simulink model "ControlDataSSM0709"  (R2023b)
settings: Solver=FixedStepAuto  StartTime=0.0  StopTime=inf  FixedStep=0.01  RelTol=1e-3
undefined symbols (not defined in the file): Down, Pull
libraries: simulink x39, speedgoatlib_IO691 x23, canmsglib x22, slrealtimeutilitieslib x1, slrealtimeiplib x1
(part 2 of 2)

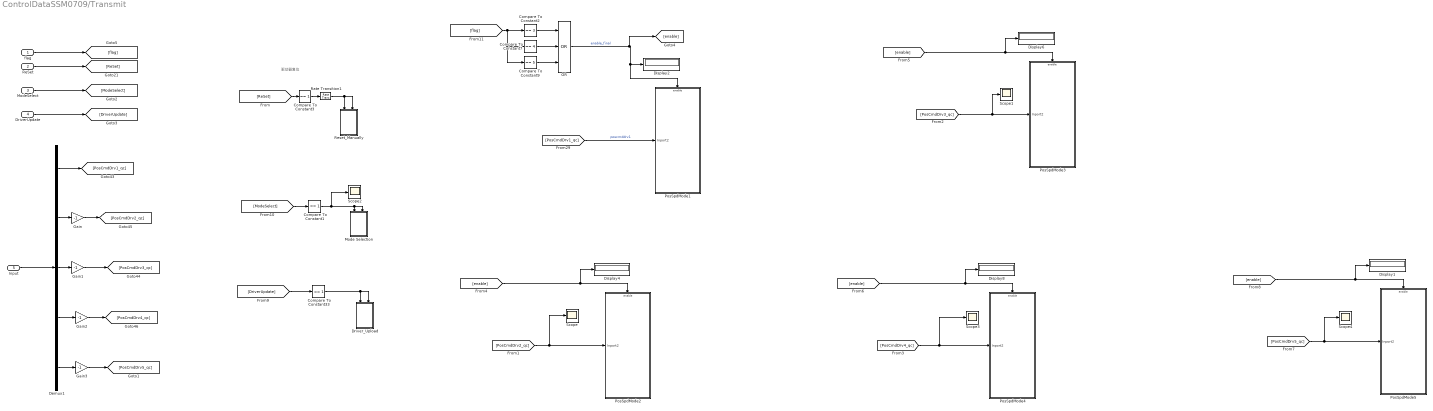
== system ControlDataSSM0709/Transmit ==
  note: 驱动器复位
  flag : Inport
  ReSet : Inport  Port=2
  ModeSelect : Inport  Port=3
  DriverUpdate : Inport  Port=4
  Input : Inport  Port=5
  Compare To Constant1 : simulink/Logic and Bit Operations/Compare To Constant  relop===  const=1  OutDataTypeStr=boolean
  Compare To Constant2 : simulink/Logic and Bit Operations/Compare To Constant  relop===  const=3  OutDataTypeStr=boolean
  Compare To Constant3 : simulink/Logic and Bit Operations/Compare To Constant  relop===  const=1  OutDataTypeStr=boolean
  Compare To Constant33 : simulink/Logic and Bit Operations/Compare To Constant  relop===  const=1  OutDataTypeStr=boolean
  Compare To Constant7 : simulink/Logic and Bit Operations/Compare To Constant  relop===  const=4  OutDataTypeStr=boolean
  Compare To Constant9 : simulink/Logic and Bit Operations/Compare To Constant  relop===  const=5  OutDataTypeStr=boolean
  Demux1 : Demux  Outputs=5
  Display{1..2,4,6,8} (5 alike) : Display
  Driver_Upload : Subsystem
  Gain{,1..3} (4 alike) : Gain  Gain=-1
  Mode Selection : Subsystem  ScheduleAs=Aperiodic partition  PartitionName=TEMP_PRECOMP_PARTITION_NAME_MessageTriggeredSubsystem
  OR : Logic  Operator=OR  Inputs=3  IconShape=distinctive  AllPortsSameDT=off  OutDataTypeStr=boolean
  PosSpdMode1 : Subsystem
  PosSpdMode2 : Subsystem
  PosSpdMode3 : Subsystem
  PosSpdMode4 : Subsystem
  PosSpdMode5 : Subsystem
  Rate Transition1 : RateTransition  OutPortSampleTime=1
  Reset_Manually : Subsystem
  Scope{,1..4} (5 alike) : Scope
  wires:
  Compare To Constant1/1 -> Mode Selection/Trigger, Mode Selection/Enable, Scope2/1
  OR/1 -> [enable], PosSpdMode1/Enable, Display2/1  "enable_final"
  [ReSet] -> Compare To Constant3/1
  Compare To Constant3/1 -> Rate Transition1/1
  Rate Transition1/1 -> Reset_Manually/Trigger, Reset_Manually/Enable
  Demux1/1 -> [PosCmdDrv1_qc]
  Demux1/3 -> Gain1/1
  Demux1/4 -> Gain2/1
  Input/1 -> Demux1/1
  Demux1/2 -> Gain/1
  ReSet/1 -> [ReSet]
  [enable] -> Display4/1, PosSpdMode2/Enable
  [enable] -> Display6/1, PosSpdMode3/Enable
  [enable] -> Display8/1, PosSpdMode4/Enable
  Compare To Constant33/1 -> Driver_Upload/Trigger, Driver_Upload/Enable
  Gain/1 -> [PosCmdDrv2_qc]
  Gain1/1 -> [PosCmdDrv3_qc]
  Gain2/1 -> [PosCmdDrv4_qc]
  [PosCmdDrv1_qc] -> PosSpdMode1/1(Inport2)  "poscmddrv1"
  [PosCmdDrv3_qc] -> Scope1/1, PosSpdMode3/1(Inport2)
  [PosCmdDrv2_qc] -> Scope/1, PosSpdMode2/1(Inport2)
  [PosCmdDrv4_qc] -> Scope3/1, PosSpdMode4/1(Inport2)
  [enable] -> Display1/1, PosSpdMode5/Enable
  [PosCmdDrv5_qc] -> Scope4/1, PosSpdMode5/1(Inport2)
  Demux1/5 -> Gain3/1
  Gain3/1 -> [PosCmdDrv5_qc]
  ModeSelect/1 -> [ModeSelect]
  DriverUpdate/1 -> [DriverUpdate]
  [ModeSelect] -> Compare To Constant1/1
  [DriverUpdate] -> Compare To Constant33/1
  flag/1 -> [flag]
  [flag] -> Compare To Constant9/1, Compare To Constant7/1, Compare To Constant2/1
  Compare To Constant2/1 -> OR/1
  Compare To Constant7/1 -> OR/2
  Compare To Constant9/1 -> OR/3

== system ControlDataSSM0709/Displacement_mode_flag=2/Subsystem1 ==
  position_in : Inport
  Enable : EnablePort
  position_out : Outport
  wires:
  position_in/1 -> position_out/1

== system ControlDataSSM0709/Displacement_mode_flag=2/Subsystem2 ==
  position_in : Inport
  Enable : EnablePort
  position_out : Outport
  wires:
  position_in/1 -> position_out/1

== system ControlDataSSM0709/Displacement_mode_flag=2/Subsystem3 ==
  position_in : Inport
  Enable : EnablePort
  position_out : Outport
  wires:
  position_in/1 -> position_out/1

== system ControlDataSSM0709/Displacement_mode_flag=2/Subsystem5 ==
  position_in : Inport
  Enable : EnablePort
  position_out : Outport
  wires:
  position_in/1 -> position_out/1

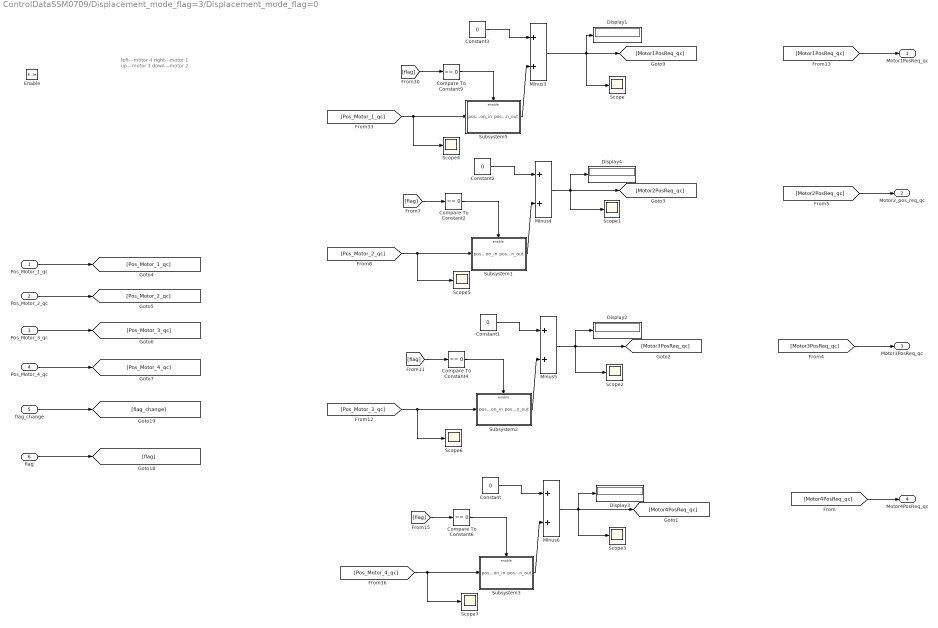
== system ControlDataSSM0709/Displacement_mode_flag=3/Displacement_mode_flag=0 ==
  note: left---motor 4
      | right---motor 1
      | up---motor 3
      | down---motor 2
  Pos_Motor_1_qc : Inport
  Pos_Motor_2_qc : Inport  Port=2
  Pos_Motor_3_qc : Inport  Port=3
  Pos_Motor_4_qc : Inport  Port=4
  flag_change : Inport  Port=5
  flag : Inport  Port=6
  Enable : EnablePort
  Compare To Constant{2,4,6,9} (4 alike) : simulink/Logic and Bit Operations/Compare To Constant  relop===  const=0  OutDataTypeStr=boolean
  Constant{,1..3} (4 alike) : Constant  Value=0
  Display{1..4} (4 alike) : Display
  Minus{3..6} (4 alike) : Sum
  Scope{,1..7} (8 alike) : Scope
  Subsystem1 : Subsystem
  Subsystem2 : Subsystem
  Subsystem3 : Subsystem
  Subsystem5 : Subsystem
  Motor1PosReq_qc : Outport
  Motor2_pos_req_qc : Outport  Port=2
  Motor3PosReq_qc : Outport  Port=3
  Motor4PosReq_qc : Outport  Port=4
  wires:
  Pos_Motor_4_qc/1 -> [Pos_Motor_4_qc]
  Pos_Motor_3_qc/1 -> [Pos_Motor_3_qc]
  Pos_Motor_2_qc/1 -> [Pos_Motor_2_qc]
  Pos_Motor_1_qc/1 -> [Pos_Motor_1_qc]
  flag/1 -> [flag]
  flag_change/1 -> [flag_change]
  [Pos_Motor_1_qc] -> Scope4/1, Subsystem5/1(position_in)
  [flag] -> Compare To Constant9/1
  Compare To Constant9/1 -> Subsystem5/Enable
  Constant3/1 -> Minus3/1
  Minus3/1 -> [Motor1PosReq_qc], Scope/1, Display1/1
  Subsystem5/1(position_out) -> Minus3/2
  Constant2/1 -> Minus4/1
  Compare To Constant2/1 -> Subsystem1/Enable
  [Pos_Motor_2_qc] -> Scope5/1, Subsystem1/1(position_in)
  Minus4/1 -> [Motor2PosReq_qc], Scope1/1, Display4/1
  Subsystem1/1(position_out) -> Minus4/2
  [flag] -> Compare To Constant2/1
  [flag] -> Compare To Constant4/1
  Subsystem2/1(position_out) -> Minus5/2
  Minus5/1 -> [Motor3PosReq_qc], Scope2/1, Display2/1
  Compare To Constant4/1 -> Subsystem2/Enable
  [Pos_Motor_3_qc] -> Scope6/1, Subsystem2/1(position_in)
  Constant1/1 -> Minus5/1
  [flag] -> Compare To Constant6/1
  Subsystem3/1(position_out) -> Minus6/2
  Minus6/1 -> [Motor4PosReq_qc], Scope3/1, Display3/1
  Compare To Constant6/1 -> Subsystem3/Enable
  [Pos_Motor_4_qc] -> Scope7/1, Subsystem3/1(position_in)
  Constant/1 -> Minus6/1
  [Motor4PosReq_qc] -> Motor4PosReq_qc/1
  [Motor3PosReq_qc] -> Motor3PosReq_qc/1
  [Motor2PosReq_qc] -> Motor2_pos_req_qc/1
  [Motor1PosReq_qc] -> Motor1PosReq_qc/1

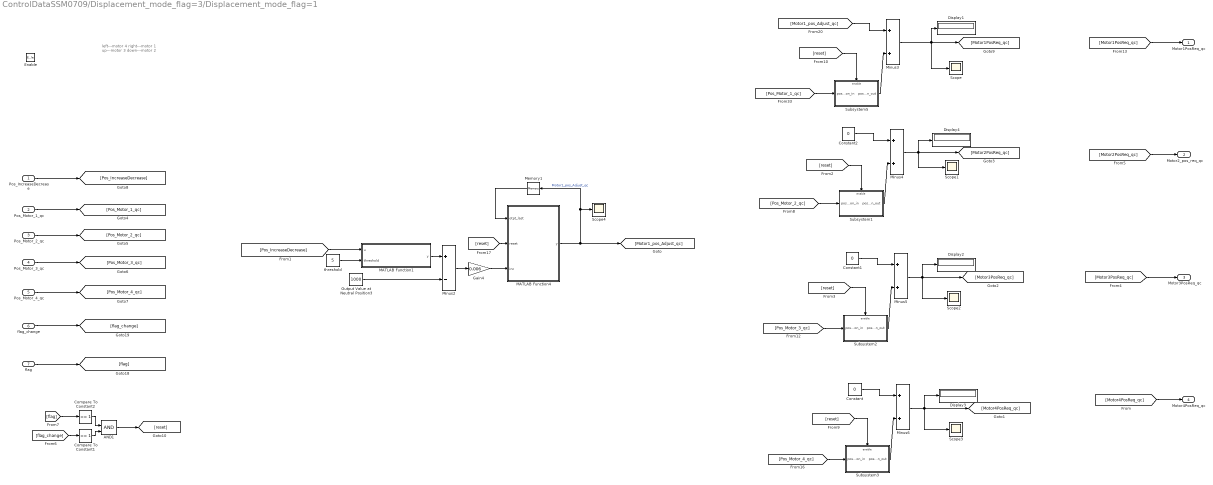
== system ControlDataSSM0709/Displacement_mode_flag=3/Displacement_mode_flag=1 ==
  note: left---motor 4
      | right---motor 1
      | up---motor 3
      | down---motor 2
  Pos_IncreaseDecrease : Inport
  Pos_Motor_1_qc : Inport  Port=2
  Pos_Motor_2_qc : Inport  Port=3
  Pos_Motor_3_qc : Inport  Port=4
  Pos_Motor_4_qc : Inport  Port=5
  flag_change : Inport  Port=6
  flag : Inport  Port=7
  Enable : EnablePort
  AND1 : Logic  IconShape=distinctive  AllPortsSameDT=off  OutDataTypeStr=boolean
  Compare To Constant1 : simulink/Logic and Bit Operations/Compare To Constant  relop===  const=1  OutDataTypeStr=boolean
  Compare To Constant2 : simulink/Logic and Bit Operations/Compare To Constant  relop===  const=1  OutDataTypeStr=boolean
  Constant : Constant  Value=0
  Constant1 : Constant  Value=0
  Constant2 : Constant  Value=0
  Display{1..4} (4 alike) : Display
  Gain4 : Gain  Gain=0.006
  MATLAB Function1 : MATLAB Function  TreatAsAtomicUnit=on
  MATLAB Function4 : MATLAB Function  TreatAsAtomicUnit=on
  Memory1 : Memory
  Minus2 : Sum  Inputs=+-
  Minus{3..6} (4 alike) : Sum
  Output Value at Neutral Position3 : Constant  Value=1000
  Scope{,1..4} (5 alike) : Scope
  Subsystem1 : Subsystem
  Subsystem2 : Subsystem
  Subsystem3 : Subsystem
  Subsystem5 : Subsystem
  threshold : Constant  Value=5
  Motor1PosReq_qc : Outport
  Motor2_pos_req_qc : Outport  Port=2
  Motor3PosReq_qc : Outport  Port=3
  Motor4PosReq_qc : Outport  Port=4
  wires:
  Minus2/1 -> Gain4/1
  [Pos_IncreaseDecrease] -> MATLAB Function1/1(u)
  MATLAB Function1/1(y) -> Minus2/1
  threshold/1 -> MATLAB Function1/2(threshold)
  Output Value at Neutral Position3/1 -> Minus2/2
  Pos_Motor_4_qc/1 -> [Pos_Motor_4_qc]
  Pos_Motor_3_qc/1 -> [Pos_Motor_3_qc]
  Pos_Motor_2_qc/1 -> [Pos_Motor_2_qc]
  Pos_Motor_1_qc/1 -> [Pos_Motor_1_qc]
  flag/1 -> [flag]
  flag_change/1 -> [flag_change]
  [Pos_Motor_1_qc] -> Subsystem5/1(position_in)
  [reset] -> Subsystem5/Enable
  [Motor1_pos_Adjust_qc] -> Minus3/1
  Minus3/1 -> [Motor1PosReq_qc], Scope/1, Display1/1
  Subsystem5/1(position_out) -> Minus3/2
  Constant2/1 -> Minus4/1
  [reset] -> Subsystem1/Enable
  [Pos_Motor_2_qc] -> Subsystem1/1(position_in)
  Minus4/1 -> [Motor2PosReq_qc], Scope1/1, Display4/1
  Subsystem1/1(position_out) -> Minus4/2
  Subsystem2/1(position_out) -> Minus5/2
  Minus5/1 -> [Motor3PosReq_qc], Scope2/1, Display2/1
  [reset] -> Subsystem2/Enable
  [Pos_Motor_3_qc] -> Subsystem2/1(position_in)
  Constant1/1 -> Minus5/1
  Subsystem3/1(position_out) -> Minus6/2
  Minus6/1 -> [Motor4PosReq_qc], Scope3/1, Display3/1
  [reset] -> Subsystem3/Enable
  [Pos_Motor_4_qc] -> Subsystem3/1(position_in)
  Constant/1 -> Minus6/1
  Gain4/1 -> MATLAB Function4/3(inc)
  Pos_IncreaseDecrease/1 -> [Pos_IncreaseDecrease]
  [Motor4PosReq_qc] -> Motor4PosReq_qc/1
  [Motor3PosReq_qc] -> Motor3PosReq_qc/1
  [Motor2PosReq_qc] -> Motor2_pos_req_qc/1
  [Motor1PosReq_qc] -> Motor1PosReq_qc/1
  [reset] -> MATLAB Function4/2(reset)
  Memory1/1 -> MATLAB Function4/1(otpt_last)
  MATLAB Function4/1(y) -> [Motor1_pos_Adjust_qc], Memory1/1, Scope4/1  "Motor1_pos_Adjust_qc"
  Compare To Constant1/1 -> AND1/2
  [flag_change] -> Compare To Constant1/1
  Compare To Constant2/1 -> AND1/1
  [flag] -> Compare To Constant2/1
  AND1/1 -> [reset]

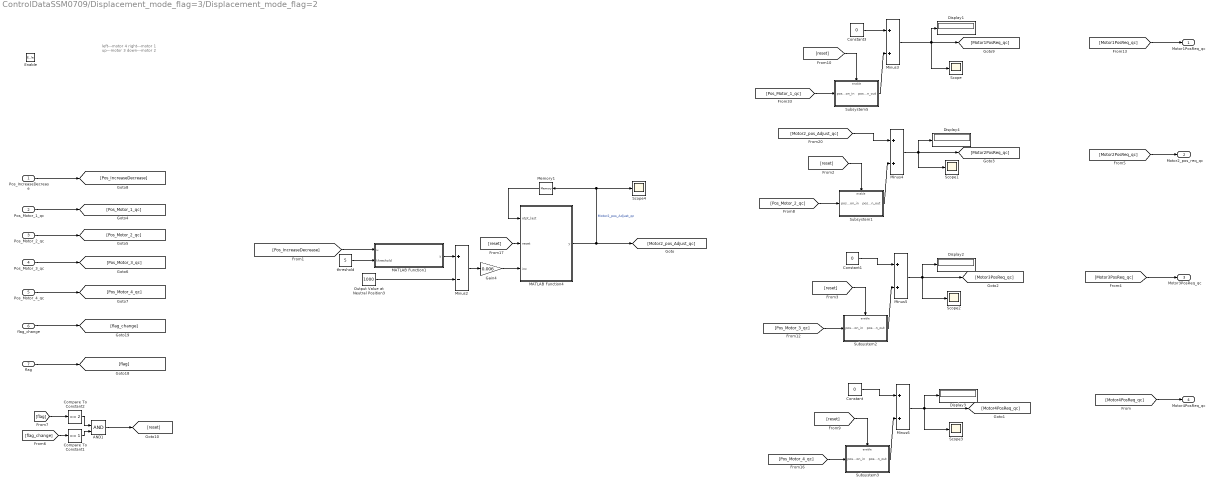
== system ControlDataSSM0709/Displacement_mode_flag=3/Displacement_mode_flag=2 ==
  note: left---motor 4
      | right---motor 1
      | up---motor 3
      | down---motor 2
  Pos_IncreaseDecrease : Inport
  Pos_Motor_1_qc : Inport  Port=2
  Pos_Motor_2_qc : Inport  Port=3
  Pos_Motor_3_qc : Inport  Port=4
  Pos_Motor_4_qc : Inport  Port=5
  flag_change : Inport  Port=6
  flag : Inport  Port=7
  Enable : EnablePort
  AND1 : Logic  IconShape=distinctive  AllPortsSameDT=off  OutDataTypeStr=boolean
  Compare To Constant1 : simulink/Logic and Bit Operations/Compare To Constant  relop===  const=1  OutDataTypeStr=boolean
  Compare To Constant2 : simulink/Logic and Bit Operations/Compare To Constant  relop===  const=2  OutDataTypeStr=boolean
  Constant : Constant  Value=0
  Constant1 : Constant  Value=0
  Constant3 : Constant  Value=0
  Display{1..4} (4 alike) : Display
  Gain4 : Gain  Gain=0.006
  MATLAB Function1 : MATLAB Function  TreatAsAtomicUnit=on
  MATLAB Function4 : MATLAB Function  TreatAsAtomicUnit=on
  Memory1 : Memory
  Minus2 : Sum  Inputs=+-
  Minus{3..6} (4 alike) : Sum
  Output Value at Neutral Position3 : Constant  Value=1000
  Scope{,1..4} (5 alike) : Scope
  Subsystem1 : Subsystem
  Subsystem2 : Subsystem
  Subsystem3 : Subsystem
  Subsystem5 : Subsystem
  threshold : Constant  Value=5
  Motor1PosReq_qc : Outport
  Motor2_pos_req_qc : Outport  Port=2
  Motor3PosReq_qc : Outport  Port=3
  Motor4PosReq_qc : Outport  Port=4
  wires:
  Minus2/1 -> Gain4/1
  [Pos_IncreaseDecrease] -> MATLAB Function1/1(u)
  MATLAB Function1/1(y) -> Minus2/1
  threshold/1 -> MATLAB Function1/2(threshold)
  Output Value at Neutral Position3/1 -> Minus2/2
  Pos_Motor_4_qc/1 -> [Pos_Motor_4_qc]
  Pos_Motor_3_qc/1 -> [Pos_Motor_3_qc]
  Pos_Motor_2_qc/1 -> [Pos_Motor_2_qc]
  Pos_Motor_1_qc/1 -> [Pos_Motor_1_qc]
  flag/1 -> [flag]
  flag_change/1 -> [flag_change]
  [Pos_Motor_1_qc] -> Subsystem5/1(position_in)
  [reset] -> Subsystem5/Enable
  Minus3/1 -> [Motor1PosReq_qc], Scope/1, Display1/1
  Subsystem5/1(position_out) -> Minus3/2
  [Motor2_pos_Adjust_qc] -> Minus4/1
  [reset] -> Subsystem1/Enable
  [Pos_Motor_2_qc] -> Subsystem1/1(position_in)
  Minus4/1 -> [Motor2PosReq_qc], Scope1/1, Display4/1
  Subsystem1/1(position_out) -> Minus4/2
  Subsystem2/1(position_out) -> Minus5/2
  Minus5/1 -> [Motor3PosReq_qc], Scope2/1, Display2/1
  [reset] -> Subsystem2/Enable
  [Pos_Motor_3_qc] -> Subsystem2/1(position_in)
  Constant1/1 -> Minus5/1
  Subsystem3/1(position_out) -> Minus6/2
  Minus6/1 -> [Motor4PosReq_qc], Scope3/1, Display3/1
  [reset] -> Subsystem3/Enable
  [Pos_Motor_4_qc] -> Subsystem3/1(position_in)
  Constant/1 -> Minus6/1
  Gain4/1 -> MATLAB Function4/3(inc)
  Pos_IncreaseDecrease/1 -> [Pos_IncreaseDecrease]
  [Motor4PosReq_qc] -> Motor4PosReq_qc/1
  [Motor3PosReq_qc] -> Motor3PosReq_qc/1
  [Motor2PosReq_qc] -> Motor2_pos_req_qc/1
  [Motor1PosReq_qc] -> Motor1PosReq_qc/1
  Constant3/1 -> Minus3/1
  Compare To Constant1/1 -> AND1/2
  [flag_change] -> Compare To Constant1/1
  Compare To Constant2/1 -> AND1/1
  [flag] -> Compare To Constant2/1
  AND1/1 -> [reset]
  [reset] -> MATLAB Function4/2(reset)
  Memory1/1 -> MATLAB Function4/1(otpt_last)
  MATLAB Function4/1(y) -> Scope4/1, Memory1/1, [Motor2_pos_Adjust_qc]  "Motor2_pos_Adjust_qc"

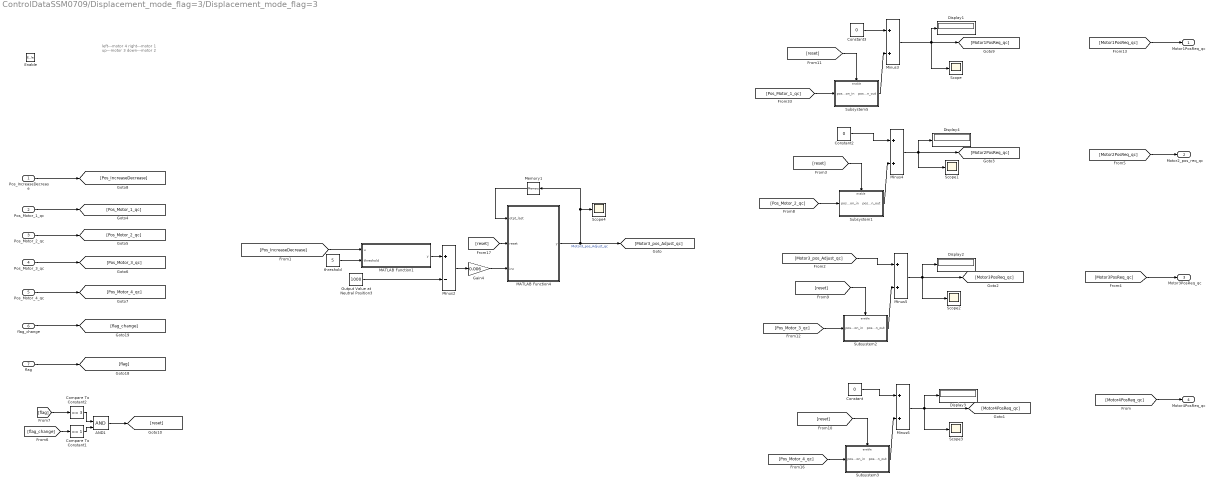
== system ControlDataSSM0709/Displacement_mode_flag=3/Displacement_mode_flag=3 ==
  note: left---motor 4
      | right---motor 1
      | up---motor 3
      | down---motor 2
  Pos_IncreaseDecrease : Inport
  Pos_Motor_1_qc : Inport  Port=2
  Pos_Motor_2_qc : Inport  Port=3
  Pos_Motor_3_qc : Inport  Port=4
  Pos_Motor_4_qc : Inport  Port=5
  flag_change : Inport  Port=6
  flag : Inport  Port=7
  Enable : EnablePort
  AND1 : Logic  IconShape=distinctive  AllPortsSameDT=off  OutDataTypeStr=boolean
  Compare To Constant1 : simulink/Logic and Bit Operations/Compare To Constant  relop===  const=1  OutDataTypeStr=boolean
  Compare To Constant2 : simulink/Logic and Bit Operations/Compare To Constant  relop===  const=3  OutDataTypeStr=boolean
  Constant : Constant  Value=0
  Constant2 : Constant  Value=0
  Constant3 : Constant  Value=0
  Display{1..4} (4 alike) : Display
  Gain4 : Gain  Gain=0.006
  MATLAB Function1 : MATLAB Function  TreatAsAtomicUnit=on
  MATLAB Function4 : MATLAB Function  TreatAsAtomicUnit=on
  Memory1 : Memory
  Minus2 : Sum  Inputs=+-
  Minus{3..6} (4 alike) : Sum
  Output Value at Neutral Position3 : Constant  Value=1000
  Scope{,1..4} (5 alike) : Scope
  Subsystem1 : Subsystem
  Subsystem2 : Subsystem
  Subsystem3 : Subsystem
  Subsystem5 : Subsystem
  threshold : Constant  Value=5
  Motor1PosReq_qc : Outport
  Motor2_pos_req_qc : Outport  Port=2
  Motor3PosReq_qc : Outport  Port=3
  Motor4PosReq_qc : Outport  Port=4
  wires:
  Minus2/1 -> Gain4/1
  [Pos_IncreaseDecrease] -> MATLAB Function1/1(u)
  MATLAB Function1/1(y) -> Minus2/1
  threshold/1 -> MATLAB Function1/2(threshold)
  Output Value at Neutral Position3/1 -> Minus2/2
  Pos_Motor_4_qc/1 -> [Pos_Motor_4_qc]
  Pos_Motor_3_qc/1 -> [Pos_Motor_3_qc]
  Pos_Motor_2_qc/1 -> [Pos_Motor_2_qc]
  Pos_Motor_1_qc/1 -> [Pos_Motor_1_qc]
  flag/1 -> [flag]
  flag_change/1 -> [flag_change]
  [Pos_Motor_1_qc] -> Subsystem5/1(position_in)
  [reset] -> Subsystem5/Enable
  Minus3/1 -> [Motor1PosReq_qc], Scope/1, Display1/1
  Subsystem5/1(position_out) -> Minus3/2
  Constant2/1 -> Minus4/1
  [reset] -> Subsystem1/Enable
  [Pos_Motor_2_qc] -> Subsystem1/1(position_in)
  Minus4/1 -> [Motor2PosReq_qc], Scope1/1, Display4/1
  Subsystem1/1(position_out) -> Minus4/2
  Subsystem2/1(position_out) -> Minus5/2
  Minus5/1 -> [Motor3PosReq_qc], Scope2/1, Display2/1
  [reset] -> Subsystem2/Enable
  [Pos_Motor_3_qc] -> Subsystem2/1(position_in)
  [Motor3_pos_Adjust_qc] -> Minus5/1
  Subsystem3/1(position_out) -> Minus6/2
  Minus6/1 -> [Motor4PosReq_qc], Scope3/1, Display3/1
  [reset] -> Subsystem3/Enable
  [Pos_Motor_4_qc] -> Subsystem3/1(position_in)
  Constant/1 -> Minus6/1
  Gain4/1 -> MATLAB Function4/3(inc)
  Pos_IncreaseDecrease/1 -> [Pos_IncreaseDecrease]
  [Motor4PosReq_qc] -> Motor4PosReq_qc/1
  [Motor3PosReq_qc] -> Motor3PosReq_qc/1
  [Motor2PosReq_qc] -> Motor2_pos_req_qc/1
  [Motor1PosReq_qc] -> Motor1PosReq_qc/1
  Constant3/1 -> Minus3/1
  Compare To Constant1/1 -> AND1/2
  [flag_change] -> Compare To Constant1/1
  [flag] -> Compare To Constant2/1
  Compare To Constant2/1 -> AND1/1
  AND1/1 -> [reset]
  [reset] -> MATLAB Function4/2(reset)
  Memory1/1 -> MATLAB Function4/1(otpt_last)
  MATLAB Function4/1(y) -> Scope4/1, Memory1/1, [Motor3_pos_Adjust_qc]  "Motor3_pos_Adjust_qc"

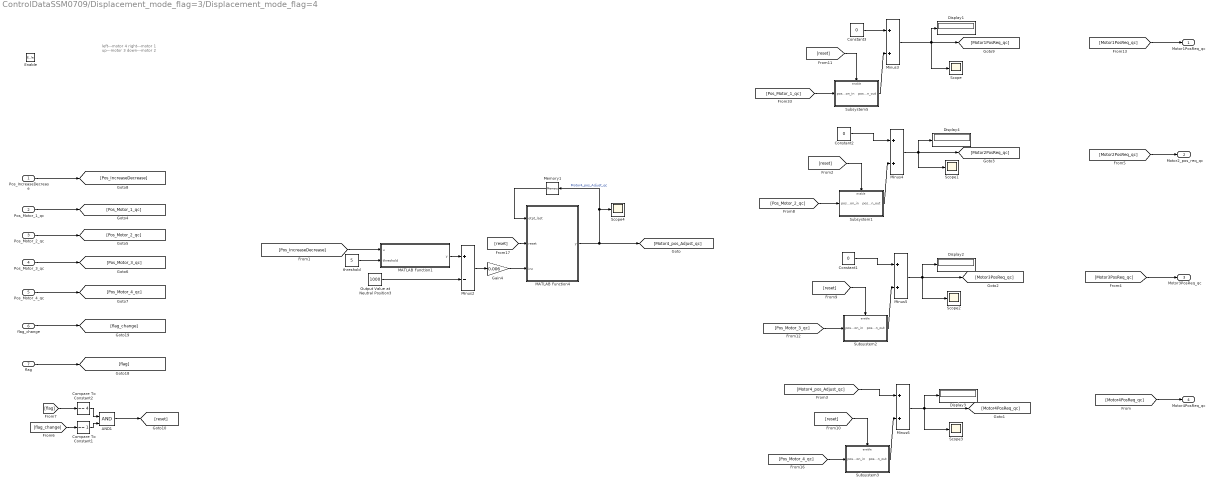
== system ControlDataSSM0709/Displacement_mode_flag=3/Displacement_mode_flag=4 ==
  note: left---motor 4
      | right---motor 1
      | up---motor 3
      | down---motor 2
  Pos_IncreaseDecrease : Inport
  Pos_Motor_1_qc : Inport  Port=2
  Pos_Motor_2_qc : Inport  Port=3
  Pos_Motor_3_qc : Inport  Port=4
  Pos_Motor_4_qc : Inport  Port=5
  flag_change : Inport  Port=6
  flag : Inport  Port=7
  Enable : EnablePort
  AND1 : Logic  IconShape=distinctive  AllPortsSameDT=off  OutDataTypeStr=boolean
  Compare To Constant1 : simulink/Logic and Bit Operations/Compare To Constant  relop===  const=1  OutDataTypeStr=boolean
  Compare To Constant2 : simulink/Logic and Bit Operations/Compare To Constant  relop===  const=4  OutDataTypeStr=boolean
  Constant1 : Constant  Value=0
  Constant2 : Constant  Value=0
  Constant3 : Constant  Value=0
  Display{1..4} (4 alike) : Display
  Gain4 : Gain  Gain=0.006
  MATLAB Function1 : MATLAB Function  TreatAsAtomicUnit=on
  MATLAB Function4 : MATLAB Function  TreatAsAtomicUnit=on
  Memory1 : Memory
  Minus2 : Sum  Inputs=+-
  Minus{3..6} (4 alike) : Sum
  Output Value at Neutral Position3 : Constant  Value=1000
  Scope{,1..4} (5 alike) : Scope
  Subsystem1 : Subsystem
  Subsystem2 : Subsystem
  Subsystem3 : Subsystem
  Subsystem5 : Subsystem
  threshold : Constant  Value=5
  Motor1PosReq_qc : Outport
  Motor2_pos_req_qc : Outport  Port=2
  Motor3PosReq_qc : Outport  Port=3
  Motor4PosReq_qc : Outport  Port=4
  wires:
  Constant3/1 -> Minus3/1
  [Motor1PosReq_qc] -> Motor1PosReq_qc/1
  [Motor2PosReq_qc] -> Motor2_pos_req_qc/1
  [Motor3PosReq_qc] -> Motor3PosReq_qc/1
  [Motor4PosReq_qc] -> Motor4PosReq_qc/1
  Pos_IncreaseDecrease/1 -> [Pos_IncreaseDecrease]
  Gain4/1 -> MATLAB Function4/3(inc)
  [Motor4_pos_Adjust_qc] -> Minus6/1
  [Pos_Motor_4_qc] -> Subsystem3/1(position_in)
  [reset] -> Subsystem3/Enable
  Minus6/1 -> Display3/1, Scope3/1, [Motor4PosReq_qc]
  Subsystem3/1(position_out) -> Minus6/2
  Constant1/1 -> Minus5/1
  [Pos_Motor_3_qc] -> Subsystem2/1(position_in)
  [reset] -> Subsystem2/Enable
  Minus5/1 -> Display2/1, Scope2/1, [Motor3PosReq_qc]
  Subsystem2/1(position_out) -> Minus5/2
  Subsystem1/1(position_out) -> Minus4/2
  Minus4/1 -> Display4/1, Scope1/1, [Motor2PosReq_qc]
  [Pos_Motor_2_qc] -> Subsystem1/1(position_in)
  [reset] -> Subsystem1/Enable
  Constant2/1 -> Minus4/1
  Subsystem5/1(position_out) -> Minus3/2
  Minus3/1 -> Display1/1, Scope/1, [Motor1PosReq_qc]
  [reset] -> Subsystem5/Enable
  [Pos_Motor_1_qc] -> Subsystem5/1(position_in)
  flag_change/1 -> [flag_change]
  flag/1 -> [flag]
  Pos_Motor_1_qc/1 -> [Pos_Motor_1_qc]
  Pos_Motor_2_qc/1 -> [Pos_Motor_2_qc]
  Pos_Motor_3_qc/1 -> [Pos_Motor_3_qc]
  Pos_Motor_4_qc/1 -> [Pos_Motor_4_qc]
  Output Value at Neutral Position3/1 -> Minus2/2
  threshold/1 -> MATLAB Function1/2(threshold)
  MATLAB Function1/1(y) -> Minus2/1
  [Pos_IncreaseDecrease] -> MATLAB Function1/1(u)
  Minus2/1 -> Gain4/1
  [flag_change] -> Compare To Constant1/1
  Compare To Constant2/1 -> AND1/1
  Compare To Constant1/1 -> AND1/2
  [flag] -> Compare To Constant2/1
  AND1/1 -> [reset]
  Memory1/1 -> MATLAB Function4/1(otpt_last)
  [reset] -> MATLAB Function4/2(reset)
  MATLAB Function4/1(y) -> Scope4/1, Memory1/1, [Motor4_pos_Adjust_qc]  "Motor4_pos_Adjust_qc"

== system ControlDataSSM0709/Transmit/Driver_Upload ==
  Enable : EnablePort  StatesWhenEnabling=reset
  Trigger : TriggerPort  VariantControl=(inherit)  PortDimensions=1
  CAN Pack : canmsglib/CAN Pack  CANdbFile=E:\OneDrive\OneDrive - The Chinese University of Hong Kong\文档\Research\SRIL\12nd\Experiment\Simulink\RoboModule0729.dbc  MsgList=Configuration_all  MsgName=Configuration_all  MsgIDType=Standard (11-bit identifier)  MsgIdentifier=10  MsgLength=8  Remote=off  ApplyMinMax=off  BusOutput=off  SignalInfo={'Data2','16','8','BE','unsigned','Standard','0','1','0','-Inf','Inf';'Data3','24','8','BE','unsigned','Standard','0','1','0','-Inf','Inf';'Data4','32','8','BE','unsigned','Standard','0','1','0','-Inf','Inf';'Data5','40','8','BE','unsigned','Standard','0','1','0','-Inf','Inf';'Data6','48','8','BE','unsigned','Standard','0','1','0','-Inf','Inf';'Data7','56','8','BE','unsigned','Standard','0','1','0','-Inf','Inf';'output_cycle_curvelpos','0','8','BE','unsigned','Standard','0','1','0','-Inf','Inf';'output_cycle_others','8','8','BE','unsigned','Standard','0','1','0','-Inf','Inf'}
      settings: DataFormat=CANdb specified signals
  "CAN Write " : speedgoatlib_IO691/CAN Write   moduleType=IO691  id=1  channel=1  canType=CAN (HS)  messageType=CAN (HS)  useBusIn=off  numOfMsg=1  enableInput=off  enableStatusPort=off  ts=-1  initValues=[691 1 -1 0 1 1 0 1 0 0]
      settings: SourceProductName=Simulink Real-Time: Speedgoat I/O Blockset
  Constant4 : Constant  Value=hex2dec('0x55')  OutDataTypeStr=uint8  SampleTime=-1
  Constant5 : Constant  Value=hex2dec('0x64')  OutDataTypeStr=uint8  SampleTime=-1
  Constant6 : Constant  Value=hex2dec('0x00')  OutDataTypeStr=uint8  SampleTime=-1
  wires:
  CAN Pack/1 -> "CAN Write "/1
  Constant4/1 -> CAN Pack/1, CAN Pack/3, CAN Pack/5, CAN Pack/6, CAN Pack/4, CAN Pack/2
  Constant5/1 -> CAN Pack/7
  Constant6/1 -> CAN Pack/8

== system ControlDataSSM0709/Transmit/Mode Selection ==
  Enable : EnablePort  StatesWhenEnabling=reset
  Trigger : TriggerPort  VariantControl=(inherit)  PortDimensions=1
  CAN Pack : canmsglib/CAN Pack  CANdbFile=E:\Research\SRIL\12nd\Simulink\RoboModule0729.dbc  MsgList=Mode_Selection_all  MsgName=Mode_Selection_all  MsgIDType=Standard (11-bit identifier)  MsgIdentifier=1  MsgLength=8  Remote=off  ApplyMinMax=off  BusOutput=off  SignalInfo={'Data1','8','8','BE','unsigned','Standard','0','1','0','-Inf','Inf';'Data2','16','8','BE','unsigned','Standard','0','1','0','-Inf','Inf';'Data3','24','8','BE','unsigned','Standard','0','1','0','-Inf','Inf';'Data4','32','8','BE','unsigned','Standard','0','1','0','-Inf','Inf';'Data5','40','8','BE','unsigned','Standard','0','1','0','-Inf','Inf';'Data6','48','8','BE','unsigned','Standard','0','1','0','-Inf','Inf';'Data7','56','8','BE','unsigned','Standard','0','1','0','-Inf','Inf';'Mode','0','8','BE','unsigned','Standard','0','1','0','-Inf','Inf'}
      settings: DataFormat=CANdb specified signals
  "CAN Write " : speedgoatlib_IO691/CAN Write   moduleType=IO691  id=1  channel=1  canType=CAN (HS)  messageType=CAN (HS)  useBusIn=off  numOfMsg=1  enableInput=off  enableStatusPort=off  ts=-1  initValues=[691 1 -1 0 1 1 0 1 0 0]
      settings: SourceProductName=Simulink Real-Time: Speedgoat I/O Blockset
  Constant2 : Constant  Value=hex2dec('0x55')  OutDataTypeStr=uint8  SampleTime=-1
  Mode Number1 : Constant  Value=hex2dec('0x04')  OutDataTypeStr=uint8  SampleTime=-1
  wires:
  Constant2/1 -> CAN Pack/1, CAN Pack/3, CAN Pack/5, CAN Pack/6, CAN Pack/7, CAN Pack/4, CAN Pack/2
  CAN Pack/1 -> "CAN Write "/1
  Mode Number1/1 -> CAN Pack/8

== system ControlDataSSM0709/Transmit/PosSpdMode1 ==
  note: R ated Voltage of Motor is 12 V. Supply Voltage is 24 V. Limilation of the temp_pwm is set as 2500.
  Inport2 : Inport
  Enable : EnablePort
  CAN Pack : canmsglib/CAN Pack  CANdbFile=E:\OneDrive\OneDrive - The Chinese University of Hong Kong\文档\Research\SRIL\12nd\Experiment\Simulink\RoboModule0729.dbc  MsgList=Position_Dr1  MsgName=Position_Dr1  MsgIDType=Standard (11-bit identifier)  MsgIdentifier=21  MsgLength=8  Remote=off  ApplyMinMax=off  BusOutput=off  SignalInfo={'Data2','16','8','BE','unsigned','Standard','0','1','0','-Inf','Inf';'Data3','24','8','BE','unsigned','Standard','0','1','0','-Inf','Inf';'temp_position','56','32','BE','signed','Standard','0','1','0','-Inf','Inf';'temp_pwm','8','16','BE','unsigned','Standard','0','1','0','-Inf','Inf'}
      settings: DataFormat=CANdb specified signals
  "CAN Write " : speedgoatlib_IO691/CAN Write   moduleType=IO691  id=1  channel=1  canType=CAN (HS)  messageType=CAN (HS)  useBusIn=off  numOfMsg=1  enableInput=off  enableStatusPort=off  ts=-1  initValues=[691 1 -1 0 1 1 0 1 0 0]
      settings: SourceProductName=Simulink Real-Time: Speedgoat I/O Blockset
  Constant1 : Constant  Value=5000
  Constant3 : Constant  Value=hex2dec('0x55')  OutDataTypeStr=uint8  SampleTime=-1
  wires:
  Constant3/1 -> CAN Pack/2, CAN Pack/1
  Inport2/1 -> CAN Pack/3
  Constant1/1 -> CAN Pack/4
  CAN Pack/1 -> "CAN Write "/1

== system ControlDataSSM0709/Transmit/PosSpdMode2 ==
  note: R ated Voltage of Motor is 12 V. Supply Voltage is 24 V. Limilation of the temp_pwm is set as 2500.
  Inport2 : Inport
  Enable : EnablePort
  CAN Pack : canmsglib/CAN Pack  CANdbFile=E:\Research\SRIL\12nd\Simulink\RoboModule0729.dbc  MsgList=Position_Dr2  MsgName=Position_Dr2  MsgIDType=Standard (11-bit identifier)  MsgIdentifier=37  MsgLength=8  Remote=off  ApplyMinMax=off  BusOutput=off  SignalInfo={'Data2','16','8','BE','unsigned','Standard','0','1','0','-Inf','Inf';'Data3','24','8','BE','unsigned','Standard','0','1','0','-Inf','Inf';'temp_position','56','32','BE','signed','Standard','0','1','0','-Inf','Inf';'temp_pwm','8','16','BE','unsigned','Standard','0','1','0','-Inf','Inf'}
      settings: DataFormat=CANdb specified signals
  "CAN Write " : speedgoatlib_IO691/CAN Write   moduleType=IO691  id=1  channel=1  canType=CAN (HS)  messageType=CAN (HS)  useBusIn=off  numOfMsg=1  enableInput=off  enableStatusPort=off  ts=-1  initValues=[691 1 -1 0 1 1 0 1 0 0]
      settings: SourceProductName=Simulink Real-Time: Speedgoat I/O Blockset
  Constant1 : Constant  Value=5000
  Constant3 : Constant  Value=hex2dec('0x55')  OutDataTypeStr=uint8  SampleTime=-1
  Scope : Scope
  wires:
  CAN Pack/1 -> "CAN Write "/1
  Constant3/1 -> CAN Pack/2, CAN Pack/1
  Inport2/1 -> Scope/1, CAN Pack/3
  Constant1/1 -> CAN Pack/4

== system ControlDataSSM0709/Transmit/PosSpdMode3 ==
  note: R ated Voltage of Motor is 12 V. Supply Voltage is 24 V. Limilation of the temp_pwm is set as 2500.
  Inport2 : Inport
  Enable : EnablePort
  CAN Pack : canmsglib/CAN Pack  CANdbFile=E:\OneDrive\OneDrive - The Chinese University of Hong Kong\文档\Research\SRIL\12nd\Experiment\Simulink\RoboModule0729.dbc  MsgList=Position_Dr3  MsgName=Position_Dr3  MsgIDType=Standard (11-bit identifier)  MsgIdentifier=53  MsgLength=8  Remote=off  ApplyMinMax=off  BusOutput=off  SignalInfo={'Data2','16','8','BE','unsigned','Standard','0','1','0','-Inf','Inf';'Data3','24','8','BE','unsigned','Standard','0','1','0','-Inf','Inf';'temp_position','56','32','BE','signed','Standard','0','1','0','-Inf','Inf';'temp_pwm','8','16','BE','unsigned','Standard','0','1','0','-Inf','Inf'}
      settings: DataFormat=CANdb specified signals
  "CAN Write " : speedgoatlib_IO691/CAN Write   moduleType=IO691  id=1  channel=1  canType=CAN (HS)  messageType=CAN (HS)  useBusIn=off  numOfMsg=1  enableInput=off  enableStatusPort=off  ts=-1  initValues=[691 1 -1 0 1 1 0 1 0 0]
      settings: SourceProductName=Simulink Real-Time: Speedgoat I/O Blockset
  Constant1 : Constant  Value=5000
  Constant3 : Constant  Value=hex2dec('0x55')  OutDataTypeStr=uint8  SampleTime=-1
  wires:
  CAN Pack/1 -> "CAN Write "/1
  Constant3/1 -> CAN Pack/2, CAN Pack/1
  Inport2/1 -> CAN Pack/3
  Constant1/1 -> CAN Pack/4

== system ControlDataSSM0709/Transmit/PosSpdMode4 ==
  note: R ated Voltage of Motor is 12 V. Supply Voltage is 24 V. Limilation of the temp_pwm is set as 2500.
  Inport2 : Inport
  Enable : EnablePort
  CAN Pack : canmsglib/CAN Pack  CANdbFile=E:\OneDrive\OneDrive - The Chinese University of Hong Kong\文档\Research\SRIL\12nd\Experiment\Simulink\RoboModule0729.dbc  MsgList=Position_Dr4  MsgName=Position_Dr4  MsgIDType=Standard (11-bit identifier)  MsgIdentifier=69  MsgLength=8  Remote=off  ApplyMinMax=off  BusOutput=off  SignalInfo={'Data2','16','8','BE','unsigned','Standard','0','1','0','-Inf','Inf';'Data3','24','8','BE','unsigned','Standard','0','1','0','-Inf','Inf';'temp_position','56','32','BE','signed','Standard','0','1','0','-Inf','Inf';'temp_pwm','8','16','BE','unsigned','Standard','0','1','0','-Inf','Inf'}
      settings: DataFormat=CANdb specified signals
  "CAN Write " : speedgoatlib_IO691/CAN Write   moduleType=IO691  id=1  channel=1  canType=CAN (HS)  messageType=CAN (HS)  useBusIn=off  numOfMsg=1  enableInput=off  enableStatusPort=off  ts=-1  initValues=[691 1 -1 0 1 1 0 1 0 0]
      settings: SourceProductName=Simulink Real-Time: Speedgoat I/O Blockset
  Constant1 : Constant  Value=5000
  Constant3 : Constant  Value=hex2dec('0x55')  OutDataTypeStr=uint8  SampleTime=-1
  wires:
  CAN Pack/1 -> "CAN Write "/1
  Constant3/1 -> CAN Pack/2, CAN Pack/1
  Inport2/1 -> CAN Pack/3
  Constant1/1 -> CAN Pack/4

== system ControlDataSSM0709/Transmit/PosSpdMode5 ==
  note: R ated Voltage of Motor is 12 V. Supply Voltage is 24 V. Limilation of the temp_pwm is set as 2500.
  Inport2 : Inport
  Enable : EnablePort
  CAN Pack : canmsglib/CAN Pack  CANdbFile=E:\OneDrive\OneDrive - The Chinese University of Hong Kong\文档\Research\SRIL\12nd\Experiment\Simulink\RoboModule0729.dbc  MsgList=Position_Dr5  MsgName=Position_Dr5  MsgIDType=Standard (11-bit identifier)  MsgIdentifier=85  MsgLength=8  Remote=off  ApplyMinMax=off  BusOutput=off  SignalInfo={'Data2','16','8','BE','unsigned','Standard','0','1','0','-Inf','Inf';'Data3','24','8','BE','unsigned','Standard','0','1','0','-Inf','Inf';'temp_position','56','32','BE','signed','Standard','0','1','0','-Inf','Inf';'temp_pwm','8','16','BE','unsigned','Standard','0','1','0','-Inf','Inf'}
      settings: DataFormat=CANdb specified signals
  "CAN Write " : speedgoatlib_IO691/CAN Write   moduleType=IO691  id=1  channel=1  canType=CAN (HS)  messageType=CAN (HS)  useBusIn=off  numOfMsg=1  enableInput=off  enableStatusPort=off  ts=-1  initValues=[691 1 -1 0 1 1 0 1 0 0]
      settings: SourceProductName=Simulink Real-Time: Speedgoat I/O Blockset
  Constant1 : Constant  Value=5000
  Constant3 : Constant  Value=hex2dec('0x55')  OutDataTypeStr=uint8  SampleTime=-1
  Scope : Scope
  wires:
  CAN Pack/1 -> "CAN Write "/1
  Constant3/1 -> CAN Pack/2, CAN Pack/1
  Inport2/1 -> Scope/1, CAN Pack/3
  Constant1/1 -> CAN Pack/4

== system ControlDataSSM0709/Transmit/Reset_Manually ==
  Enable : EnablePort  StatesWhenEnabling=reset
  Trigger : TriggerPort  VariantControl=(inherit)  PortDimensions=1
  CAN Pack : canmsglib/CAN Pack  CANdbFile=E:\OneDrive\OneDrive - The Chinese University of Hong Kong\文档\Research\SRIL\12nd\Experiment\Simulink\RoboModule0729.dbc  MsgList=Reset_all  MsgName=Reset_all  MsgIDType=Standard (11-bit identifier)  MsgIdentifier=0  MsgLength=8  Remote=off  ApplyMinMax=off  BusOutput=off  SignalInfo={'Data0','0','8','BE','unsigned','Standard','0','1','0','-Inf','Inf';'Data1','8','8','BE','unsigned','Standard','0','1','0','-Inf','Inf';'Data2','16','8','BE','unsigned','Standard','0','1','0','-Inf','Inf';'Data3','24','8','BE','unsigned','Standard','0','1','0','-Inf','Inf';'Data4','32','8','BE','unsigned','Standard','0','1','0','-Inf','Inf';'Data5','40','8','BE','unsigned','Standard','0','1','0','-Inf','Inf';'Data6','48','8','BE','unsigned','Standard','0','1','0','-Inf','Inf';'Data7','56','8','BE','unsigned','Standard','0','1','0','-Inf','Inf'}
      settings: DataFormat=CANdb specified signals
  "CAN Write " : speedgoatlib_IO691/CAN Write   moduleType=IO691  id=1  channel=1  canType=CAN (HS)  messageType=CAN (HS)  useBusIn=off  numOfMsg=1  enableInput=off  enableStatusPort=off  ts=-1  initValues=[691 1 -1 0 1 1 0 1 0 0]
      settings: SourceProductName=Simulink Real-Time: Speedgoat I/O Blockset
  Constant2 : Constant  Value=hex2dec('0x55')  OutDataTypeStr=uint8  SampleTime=-1
  wires:
  CAN Pack/1 -> "CAN Write "/1
  Constant2/1 -> CAN Pack/1, CAN Pack/3, CAN Pack/5, CAN Pack/6, CAN Pack/7, CAN Pack/8, CAN Pack/4, CAN Pack/2

== system ControlDataSSM0709/Displacement_mode_flag=3/Displacement_mode_flag=0/Subsystem1 ==
  position_in : Inport
  Enable : EnablePort
  position_out : Outport
  wires:
  position_in/1 -> position_out/1

== system ControlDataSSM0709/Displacement_mode_flag=3/Displacement_mode_flag=0/Subsystem2 ==
  position_in : Inport
  Enable : EnablePort
  position_out : Outport
  wires:
  position_in/1 -> position_out/1

== system ControlDataSSM0709/Displacement_mode_flag=3/Displacement_mode_flag=0/Subsystem3 ==
  position_in : Inport
  Enable : EnablePort
  position_out : Outport
  wires:
  position_in/1 -> position_out/1

== system ControlDataSSM0709/Displacement_mode_flag=3/Displacement_mode_flag=0/Subsystem5 ==
  position_in : Inport
  Enable : EnablePort
  position_out : Outport
  wires:
  position_in/1 -> position_out/1

== system ControlDataSSM0709/Displacement_mode_flag=3/Displacement_mode_flag=1/Subsystem1 ==
  position_in : Inport
  Enable : EnablePort
  position_out : Outport
  wires:
  position_in/1 -> position_out/1

== system ControlDataSSM0709/Displacement_mode_flag=3/Displacement_mode_flag=1/Subsystem2 ==
  position_in : Inport
  Enable : EnablePort
  position_out : Outport
  wires:
  position_in/1 -> position_out/1

== system ControlDataSSM0709/Displacement_mode_flag=3/Displacement_mode_flag=1/Subsystem3 ==
  position_in : Inport
  Enable : EnablePort
  position_out : Outport
  wires:
  position_in/1 -> position_out/1

== system ControlDataSSM0709/Displacement_mode_flag=3/Displacement_mode_flag=1/Subsystem5 ==
  position_in : Inport
  Enable : EnablePort
  position_out : Outport
  wires:
  position_in/1 -> position_out/1

== system ControlDataSSM0709/Displacement_mode_flag=3/Displacement_mode_flag=2/Subsystem1 ==
  position_in : Inport
  Enable : EnablePort
  position_out : Outport
  wires:
  position_in/1 -> position_out/1

== system ControlDataSSM0709/Displacement_mode_flag=3/Displacement_mode_flag=2/Subsystem2 ==
  position_in : Inport
  Enable : EnablePort
  position_out : Outport
  wires:
  position_in/1 -> position_out/1

== system ControlDataSSM0709/Displacement_mode_flag=3/Displacement_mode_flag=2/Subsystem3 ==
  position_in : Inport
  Enable : EnablePort
  position_out : Outport
  wires:
  position_in/1 -> position_out/1

== system ControlDataSSM0709/Displacement_mode_flag=3/Displacement_mode_flag=2/Subsystem5 ==
  position_in : Inport
  Enable : EnablePort
  position_out : Outport
  wires:
  position_in/1 -> position_out/1

== system ControlDataSSM0709/Displacement_mode_flag=3/Displacement_mode_flag=3/Subsystem1 ==
  position_in : Inport
  Enable : EnablePort
  position_out : Outport
  wires:
  position_in/1 -> position_out/1

== system ControlDataSSM0709/Displacement_mode_flag=3/Displacement_mode_flag=3/Subsystem2 ==
  position_in : Inport
  Enable : EnablePort
  position_out : Outport
  wires:
  position_in/1 -> position_out/1

== system ControlDataSSM0709/Displacement_mode_flag=3/Displacement_mode_flag=3/Subsystem3 ==
  position_in : Inport
  Enable : EnablePort
  position_out : Outport
  wires:
  position_in/1 -> position_out/1

== system ControlDataSSM0709/Displacement_mode_flag=3/Displacement_mode_flag=3/Subsystem5 ==
  position_in : Inport
  Enable : EnablePort
  position_out : Outport
  wires:
  position_in/1 -> position_out/1

== system ControlDataSSM0709/Displacement_mode_flag=3/Displacement_mode_flag=4/Subsystem1 ==
  position_in : Inport
  Enable : EnablePort
  position_out : Outport
  wires:
  position_in/1 -> position_out/1

== system ControlDataSSM0709/Displacement_mode_flag=3/Displacement_mode_flag=4/Subsystem2 ==
  position_in : Inport
  Enable : EnablePort
  position_out : Outport
  wires:
  position_in/1 -> position_out/1

== system ControlDataSSM0709/Displacement_mode_flag=3/Displacement_mode_flag=4/Subsystem3 ==
  position_in : Inport
  Enable : EnablePort
  position_out : Outport
  wires:
  position_in/1 -> position_out/1

== system ControlDataSSM0709/Displacement_mode_flag=3/Displacement_mode_flag=4/Subsystem5 ==
  position_in : Inport
  Enable : EnablePort
  position_out : Outport
  wires:
  position_in/1 -> position_out/1

== matlab function ControlDataSSM0709/Displacement_mode_flag=2/RandomControlSequence ==
  settings: updateMethod=DISCRETE
  data: disMotor1 output; disMotor2 output; t input; y_axis data_store_memory; z_axis data_store_memory; disMotor3 output; disMotor4 output; ins output; gain input; zMotor output; yMotor output
function [disMotor1,disMotor2,disMotor3,disMotor4,ins,zMotor,yMotor] = controlCmdGeneration(t,gain)
global y_axis z_axis
spdRegFactor = 0.2;
length = 5021;
retractionrFactor = 2;
tFinal = t*spdRegFactor;
ins = fix(tFinal);
if ins <= length
    yMotorOrg = y_axis(ins);
    zMotorOrg = z_axis(ins);
else
    yMotorOrg = 0;
    zMotorOrg = 0;
end

yMotor = gain*min(1, max(-1, yMotorOrg));
zMotor = gain*min(1, max(-1, zMotorOrg));

if zMotor > 0
    disMotor4 = zMotor;
    disMotor1 = -retractionrFactor*zMotor;
else
    disMotor4 = retractionrFactor*zMotor;
    disMotor1 = -zMotor;
end

if yMotor > 0
    disMotor2 = yMotor;
    disMotor3 = -retractionrFactor*yMotor;
else
    disMotor2 = retractionrFactor*yMotor;
    disMotor3 = -yMotor;
end

end

== matlab function ControlDataSSM0709/MATLAB Function1 ==
  data: y output; u_out output; u input; u_last input
function [y,u_out] = fcn(u,u_last)
if abs(u-u_last)>20
    y = 1;
else
    y = 0;
end
u_out = u;

== matlab function ControlDataSSM0709/MATLAB Function2 ==
  data: y output; u_out output; u input; u_last input
function [y,u_out] = fcn(u,u_last)
if abs(u-u_last)>20
    y = 1;
else
    y = 0;
end
u_out = u;

== matlab function ControlDataSSM0709/Initial_flag=1/RandomControlSequence ==
  settings: updateMethod=DISCRETE
  data: u output; force_meas input; F_min input; F_max input; step input
function u = tension_control(force_meas,F_min,F_max,step)
    u_pull = step; % small constant torque or velocity
    u_relax = -step;
    
    if force_meas < F_min
        u = u_pull;
    elseif force_meas > F_max
        u = u_relax;
    else
        u = 0; % hold
    end
end

== matlab function ControlDataSSM0709/Initial_flag=1/RandomControlSequence1 ==
  settings: updateMethod=DISCRETE
  data: u output; force_meas input; F_min input; F_max input; step input
function u = tension_control(force_meas,F_min,F_max,step)
    u_pull = step; % small constant torque or velocity
    u_relax = -step;
    
    if force_meas < F_min
        u = u_pull;
    elseif force_meas > F_max
        u = u_relax;
    else
        u = 0; % hold
    end
end

== matlab function ControlDataSSM0709/Initial_flag=1/RandomControlSequence2 ==
  settings: updateMethod=DISCRETE
  data: u output; force_meas input; F_min input; F_max input; step input
function u = tension_control(force_meas,F_min,F_max,step)
    u_pull = step; % small constant torque or velocity
    u_relax = -step;
    
    if force_meas < F_min
        u = u_pull;
    elseif force_meas > F_max
        u = u_relax;
    else
        u = 0; % hold
    end
end

== matlab function ControlDataSSM0709/Initial_flag=1/RandomControlSequence3 ==
  settings: updateMethod=DISCRETE
  data: u output; force_meas input; F_min input; F_max input; step input
function u = tension_control(force_meas,F_min,F_max,step)
    u_pull = step; % small constant torque or velocity
    u_relax = -step;
    
    if force_meas < F_min
        u = u_pull;
    elseif force_meas > F_max
        u = u_relax;
    else
        u = 0; % hold
    end
end

== matlab function ControlDataSSM0709/Subsystem/MATLAB Function5 ==
  data: y output; u input; threshold input
function y = noise_reduction(u,threshold)
if abs(u - 1000) > threshold
    y = u;
else
    y = 1000;
end

== matlab function ControlDataSSM0709/Displacement_mode_flag=3/Displacement_mode_flag=1/MATLAB Function1 ==
  data: y output; u input; threshold input
function y = noise_reduction(u,threshold)
if abs(u - 1000) > threshold
    y = u;
else
    y = 1000;
end

== matlab function ControlDataSSM0709/Displacement_mode_flag=3/Displacement_mode_flag=2/MATLAB Function1 ==
  data: y output; u input; threshold input
function y = noise_reduction(u,threshold)
if abs(u - 1000) > threshold
    y = u;
else
    y = 1000;
end

== stateflow chart ControlDataSSM0709/Displacement_mode_flag=3/Chart2 ==
  settings: sampleTime=0.001
  state b [parallel]
    settings: executionOrder=1
    state LeftMotor4
      during:flag_direction=4;
    state RightMotor1
      during:flag_direction=1;
    state off
      during:flag_direction=0;
    state UpMotor3
      during:flag_direction=3;
    state DownMotor2
      during:flag_direction=2;
    LeftMotor4 -> off : [duration(LeftMotor4_RightMotor1 < 400) > 1|| reset > 0]
    off -> LeftMotor4 [order 1] : [duration(LeftMotor4_RightMotor1 < 400) > 1]
    RightMotor1 -> off : [duration(LeftMotor4_RightMotor1 > 1600) > 1 || reset > 0]
    (default) -> off
    off -> RightMotor1 [order 2] : [duration(LeftMotor4_RightMotor1 > 1600) > 1]
    off -> DownMotor2 [order 4] : [duration(UpMotor3_DownMotor2 > 1600) > 1]
    DownMotor2 -> off : [duration(UpMotor3_DownMotor2 > 1600) > 1 || reset > 0]
    off -> UpMotor3 [order 3] : [duration(UpMotor3_DownMotor2 < 400) > 1]
    UpMotor3 -> off : [duration(UpMotor3_DownMotor2 < 400) > 1 || reset > 0]
  data: flag_direction output double; LeftMotor4_RightMotor1 input double; UpMotor3_DownMotor2 input double; reset input boolean

== matlab function ControlDataSSM0709/Displacement_mode_flag=3/Displacement_mode_flag=3/MATLAB Function1 ==
  data: y output; u input; threshold input
function y = noise_reduction(u,threshold)
if abs(u - 1000) > threshold
    y = u;
else
    y = 1000;
end

== matlab function ControlDataSSM0709/Displacement_mode_flag=3/Displacement_mode_flag=4/MATLAB Function1 ==
  data: y output; u input; threshold input
function y = noise_reduction(u,threshold)
if abs(u - 1000) > threshold
    y = u;
else
    y = 1000;
end

== matlab function ControlDataSSM0709/MATLAB Function11 ==
  data: y output; u input; u_last input
function y = fcn(u,u_last)
if abs(u-u_last)>200
    y = u_last;
else
    y = u;
end

== matlab function ControlDataSSM0709/Displacement_mode_flag=3/Displacement_mode_flag=1/MATLAB Function4 ==
  data: y output; otpt_last input; reset input; inc input
function y = noise_reduction(otpt_last,reset,inc)
if reset > 0.5
    aa = 0;
else
    aa = otpt_last;
end
y = aa + inc;

== matlab function ControlDataSSM0709/Displacement_mode_flag=3/Displacement_mode_flag=2/MATLAB Function4 ==
  data: y output; otpt_last input; reset input; inc input
function y = noise_reduction(otpt_last,reset,inc)
if reset > 0.5
    aa = 0;
else
    aa = otpt_last;
end
y = aa + inc;

== matlab function ControlDataSSM0709/Displacement_mode_flag=3/Displacement_mode_flag=3/MATLAB Function4 ==
  data: y output; otpt_last input; reset input; inc input
function y = noise_reduction(otpt_last,reset,inc)
if reset > 0.5
    aa = 0;
else
    aa = otpt_last;
end
y = aa + inc;

== matlab function ControlDataSSM0709/Displacement_mode_flag=3/Displacement_mode_flag=4/MATLAB Function4 ==
  data: y output; otpt_last input; reset input; inc input
function y = noise_reduction(otpt_last,reset,inc)
if reset > 0.5
    aa = 0;
else
    aa = otpt_last;
end
y = aa + inc;

== matlab function ControlDataSSM0709/Subsystem/MATLAB Function4 ==
  data: y output; otpt_last input; inc input
function y = noise_reduction(otpt_last,inc)
    aa = otpt_last;
y = aa + inc;

== stateflow chart ControlDataSSM0709/Chart1 ==
  settings: sampleTime=0.001
  note: Operation logic: The initial flag is 0. Imitating the operation logic of the drone, long press the H switch for 5 seconds, the flag changes to 1, and the system starts. Long press again for 5 seconds, and the flag changes back to 0.
  state b [parallel]
    settings: executionOrder=1
    state off
      during:flag=0;
    state ModeSelection
      during:flag=1;
    state FeedbackEnable
      during:flag=2;
    state Initialization_Mode
      during:flag=3;
    state RandomCrt
      during:flag=4;
    state IndividualAdjust
      during:flag=5;
    RandomCrt -> off [order 3] : [Switch_E_Change>0]
    Initialization_Mode -> off [order 4] : [Switch_E_Change>0]
    FeedbackEnable -> off [order 2] : [Switch_E_Change>0]
    ModeSelection -> off [order 3] : [Switch_E_Change>0]
    FeedbackEnable -> Initialization_Mode [order 1] : [Switch_A_Change > 0]
    Initialization_Mode -> RandomCrt [order 3] : [Switch_B_Change > 0]
    ModeSelection -> off [order 1] : [duration(Switch_H > 1000) > 3]
    ModeSelection -> FeedbackEnable [order 2] : after(1,sec)
    (default) -> off
    RandomCrt -> Initialization_Mode [order 1] : [Switch_B_Change > 0]
    off -> ModeSelection : [duration(Switch_H > 1000) > 3]
    Initialization_Mode -> FeedbackEnable [order 2] : [Switch_A_Change > 0]
    FeedbackEnable -> IndividualAdjust [order 3] : [Switch_C_Change > 0]
    IndividualAdjust -> Initialization_Mode [order 1] : [Switch_D_Change > 0]
    Initialization_Mode -> IndividualAdjust [order 1] : [Switch_D_Change > 0]
    IndividualAdjust -> off [order 3] : [Switch_E_Change>0]
    IndividualAdjust -> RandomCrt [order 2] : [Switch_C_Change > 0]
    RandomCrt -> IndividualAdjust [order 2] : [Switch_C_Change > 0]
  data: flag output double; Switch_A_Change input double; Switch_H input double; Switch_B_Change input double; Switch_C_Change input double; Switch_D_Change input double; Switch_E_Change input double

== matlab function ControlDataSSM0709/MATLAB Function12 ==
  data: y output; u_out output; u input; u_last input
function [y,u_out] = fcn(u,u_last)
if abs(u-u_last)>20
    y = 1;
else
    y = 0;
end
u_out = u;

== matlab function ControlDataSSM0709/MATLAB Function14 ==
  data: y output; u_out output; u input; u_last input
function [y,u_out] = fcn(u,u_last)
if abs(u-u_last)>20
    y = 1;
else
    y = 0;
end
u_out = u;

== matlab function ControlDataSSM0709/MATLAB Function15 ==
  data: y output; u_out output; u input; u_last input
function [y,u_out] = fcn(u,u_last)
if abs(u-u_last)>20
    y = 1;
else
    y = 0;
end
u_out = u;

== matlab function ControlDataSSM0709/MATLAB Function16 ==
  data: y output; u_out output; u input; u_last input
function [y,u_out] = fcn(u,u_last)
if abs(u-u_last)>20
    y = 1;
else
    y = 0;
end
u_out = u;

== matlab function ControlDataSSM0709/MATLAB Function5 ==
  data: y output; u_out output; u input; u_last input
function [y,u_out] = fcn(u,u_last)
if abs(u-u_last)>20
    y = 1;
else
    y = 0;
end
u_out = u;
